simulink model "P1_1c"  (R2021b)
settings: Solver=VariableStepAuto  StartTime=0.0  StopTime=10.0  RelTol=1e-3
undefined symbols (not defined in the file or in its folder): J1, J2, J3
settings Model: Creator=mluser  LastModifiedBy=mluser

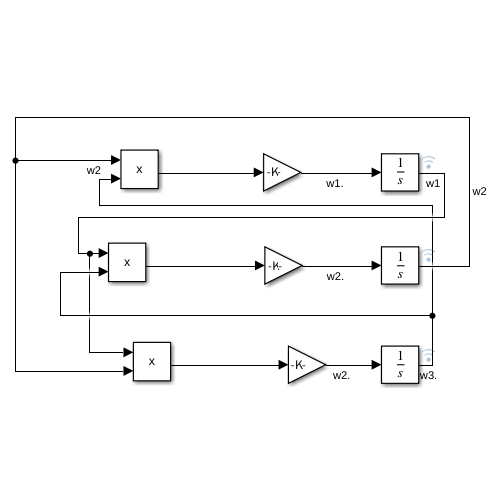
[thumbnail: Simulink's stored preview of the top-level diagram]
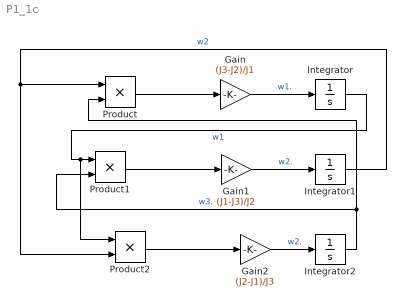
== system P1_1c ==
  Gain : Gain  Gain=(J3-J2)/J1
  Gain1 : Gain  Gain=(J1-J3)/J2
  Gain2 : Gain  Gain=(J2-J1)/J3
  Integrator : Integrator  InitialCondition=1
  Integrator1 : Integrator  InitialCondition=1
  Integrator2 : Integrator  InitialCondition=1
  Product : Product
  Product1 : Product
  Product2 : Product
  wires:
  Product/1 -> Gain/1
  Integrator1/1 -> Product/1, Product2/2  "w2"
  Gain/1 -> Integrator/1  "w1."
  Product1/1 -> Gain1/1
  Gain1/1 -> Integrator1/1  "w2."
  Integrator/1 -> Product2/1, Product1/1  "w1"
  Gain2/1 -> Integrator2/1  "w2."
  Integrator2/1 -> Product1/2, Product/2  "w3."
  Product2/1 -> Gain2/1
